simulink model "sim_localization_old"  (R2025b)
settings: Solver=ode4  StartTime=0.0  StopTime=10.0  RelTol=1e-3
values from neighbouring files (symbols this model uses):
  D = diag([0.001, 0.001, 0.0175/6, 0.0175/6, 0.0175/6, 0.0175/6*T_s, 0.0175/6*T_s].^2)    [EX_opt_1.m]    (also in init_localization.m; init_localization_template.m; script_init_localization.m)
  d = 0.165    [EX_opt_1.m]    (also in id_LEO.m; init_localization.m; init_localization_template.m; script_init_localization.m)
  d_actual = 0.164    [EX_opt_1.m]    (also in data_for_identification.mat = 0.165; init_localization.m; init_localization_template.m; script_init_localization.m)
  P_INIT_EKF = diag([0.001, 0.001, 0.0175/6, 0.0175/6, 0.0175/6, 0.0175/6*T_s, 0.0175/6*T_s].^2)    [EX_opt_1.m]    (also in init_localization.m; init_localization_template.m; script_init_localization.m)
  PHI_INIT = [0;0]    [EX_opt_1.m]    (also in data_for_identification.mat = [0 0]; id_LEO.m; init_localization.m; init_localization_template.m)
  Q_INIT = q(:,1)    [EX_opt_1.m]    (also in data_for_identification.mat = [0 0 0.463647609001]; id_LEO.m; init_localization.m = [0;0;0]; script_init_localization.m)
  r = 0.03    [EX_opt_1.m]    (also in id_LEO.m; init_localization.m; init_localization_template.m; script_init_localization.m)
  R_2 = diag([ENCODER_QUANTIZATION/6, ENCODER_QUANTIZATION/6].^2)    [EX_opt_1.m]    (also in init_localization.m = diag([ENCODER_QUANRIZATION/6,ENCODER_QUANRIZATION/6].^2); init_localization_template.m = diag([ENCODER_QUANRIZATION/6,ENCODER_QUANRIZATION/6].^2); script_init_localization.m = diag([ENCODER_QUANRIZATION/6,ENCODER_QUANRIZATION/6].^2))
  R_4 = diag([noise_std, noise_std, ENCODER_QUANTIZATION/6, ENCODER_QUANTIZATION/6].^2)    [EX_opt_1.m]    (also in init_localization.m = diag(([0.001, 0.001, ENCODER_QUANRIZATION/6,ENCODER_QUANRIZA; init_localization_template.m = diag(([0.001, 0.001, ENCODER_QUANRIZATION/6,ENCODER_QUANRIZA; script_init_localization.m = diag(([0.001, 0.001, ENCODER_QUANRIZATION/6,ENCODER_QUANRIZA)
  r_actual = 0.031    [EX_opt_1.m]    (also in data_for_identification.mat = 0.03; init_localization.m; init_localization_template.m; script_init_localization.m)
  T_s = 0.04    [EX_opt_1.m]    (also in EX_opt_2.m = Ts_values(i); data_for_identification.mat; id_LEO.m; id_template.m)
  Z_INIT_EKF = [Q_INIT_LOC; 0; 0; 0; 0]    [EX_opt_1.m]    (also in init_localization.m = [0;0;0])
settings Model: Creator=llp  LastModifiedBy=llp

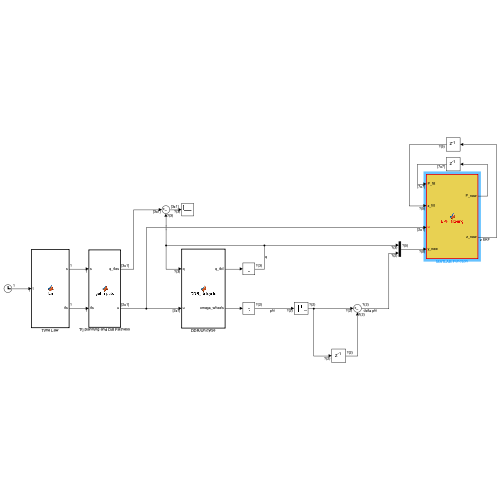
[thumbnail: Simulink's stored preview of the top-level diagram]
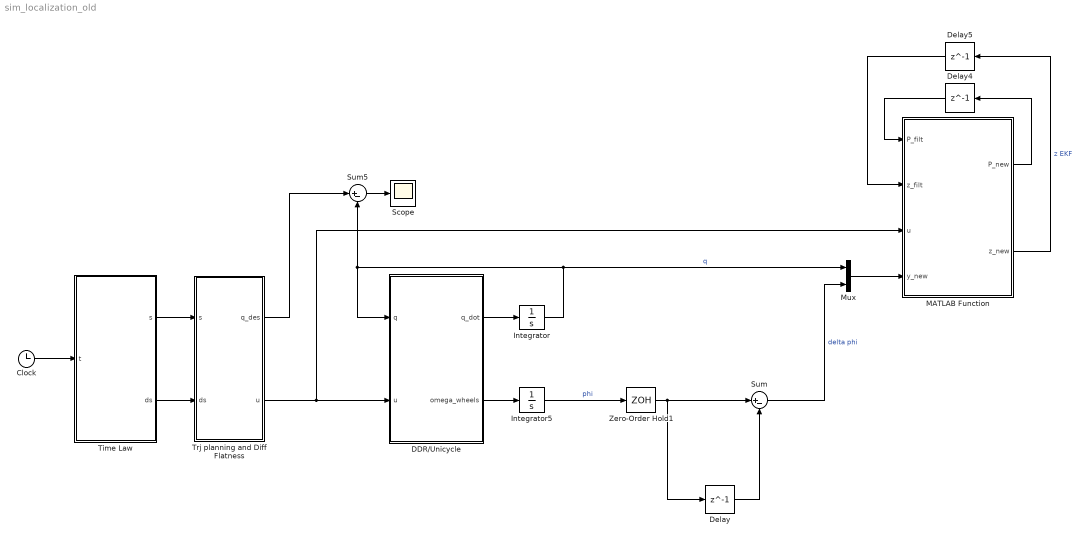
== system sim_localization_old ==
  Clock : Clock
  DDR/Unicycle : MATLAB Function  TreatAsAtomicUnit=on
  Delay : Delay  DelayLength=1  InitialCondition=[0;0]  SampleTime=T_s
  Delay4 : Delay  DelayLength=1  InitialCondition=P_INIT_EKF  SampleTime=T_s
  Delay5 : Delay  DelayLength=1  InitialCondition=Z_INIT_EKF  SampleTime=T_s
  Integrator : Integrator  InitialCondition=Q_INIT
  Integrator5 : Integrator  InitialCondition=PHI_INIT
  MATLAB Function : MATLAB Function  TreatAsAtomicUnit=on
  Mux : Mux  Inputs=2
  Scope : Scope
  Sum : Sum  Inputs=|+-
  Sum5 : Sum  Inputs=|+-
  Time Law : MATLAB Function  TreatAsAtomicUnit=on
  Trj planning and Diff Flatness : MATLAB Function  TreatAsAtomicUnit=on
  Zero-Order Hold1 : ZeroOrderHold  SampleTime=T_s
  wires:
  Integrator5/1 -> Zero-Order Hold1/1  "phi"
  Delay4/1 -> MATLAB Function/1(P_filt)
  Mux/1 -> MATLAB Function/4(y_new)
  Time Law/1(s) -> Trj planning and Diff Flatness/1(s)
  DDR/Unicycle/1(q_dot) -> Integrator/1
  Delay5/1 -> MATLAB Function/2(z_filt)
  Sum/1 -> Mux/2  "delta phi"
  Delay/1 -> Sum/2
  Sum5/1 -> Scope/1
  Integrator/1 -> Mux/1, Sum5/2, DDR/Unicycle/1(q)  "q"
  Time Law/2(ds) -> Trj planning and Diff Flatness/2(ds)
  MATLAB Function/2(z_new) -> Delay5/1  "z EKF"
  Zero-Order Hold1/1 -> Sum/1, Delay/1
  Trj planning and Diff Flatness/1(q_des) -> Sum5/1
  DDR/Unicycle/2(omega_wheels) -> Integrator5/1
  Trj planning and Diff Flatness/2(u) -> MATLAB Function/3(u), DDR/Unicycle/2(u)
  MATLAB Function/1(P_new) -> Delay4/1
  Clock/1 -> Time Law/1(t)

== matlab function sim_localization_old/Time Law ==
  data: t input; s output; ds output
function [s, ds] = fcn(t)

Ta = 0.5;
Tc = 9;

T1 = Ta;
T2 = Ta + Tc;
T3 = 2*Ta + Tc;

vc = 1/(Ta+Tc);
acc = vc/Ta;


% velocità
if t < T1
    s = 0.5*acc*t^2;
    ds = acc*t;

elseif t < T2
    s = 0.5*acc*Ta^2 + vc*(t - Ta);
    ds = vc;

elseif t < T3
    s = 0.5*acc*Ta^2 + vc*Tc + vc*(t - Ta - Tc)- 0.5*acc*(t - Ta - Tc)^2;
    ds = vc - acc*(t - Ta - Tc);

else
    s = 1;
    ds = 0;
end

== matlab function sim_localization_old/DDR//Unicycle ==
  data: q input; u input; q_dot output; omega_wheels output; d_actual parameter; r_actual parameter
function [q_dot, omega_wheels] = DDR_Unicycle(q, u, d_actual, r_actual)

theta = q(3);

v = u(1);
omega = u(2);

% ----- Cinematica unicycle -----
x_dot = v * cos(theta);
y_dot = v * sin(theta);
theta_dot = omega;

q_dot = [x_dot; y_dot; theta_dot];

% ----- Velocità ruote -----
d = d_actual;
r = r_actual;

omega_R = (v + (d/2)*omega) / r;
omega_L = (v - (d/2)*omega) / r;

omega_wheels = [omega_R; omega_L];

end

== matlab function sim_localization_old/Trj planning and Diff Flatness ==
  data: q_des output; s input; u output; ds input
function [q_des, u] = get_inputs(s, ds)

R = 0.4;
omega = 2*pi;

% ----- Traiettoria -----
x = R*sin(2*omega*s);
y = R*sin(omega*s);

% ----- Derivate rispetto a s -----
dx_s  = 2*R*omega*cos(2*omega*s);
dy_s  = R*omega*cos(omega*s);

ddx_s = -4*R*omega^2*sin(2*omega*s);
ddy_s = -R*omega^2*sin(omega*s);

% ----- Time law -----
s_dot  = ds;
s_ddot = 0;   % approx (fase a velocità costante)

% ----- Chain rule -----
dx = dx_s * s_dot;
dy = dy_s * s_dot;

ddx = ddx_s * s_dot^2 + dx_s * s_ddot;
ddy = ddy_s * s_dot^2 + dy_s * s_ddot;

% ----- Flatness -----
v = sqrt(dx^2 + dy^2);

den = dx^2 + dy^2 + 1e-6;  % evita problemi numerici
omega_u = (dx*ddy - dy*ddx) / den;

theta = atan2(dy, dx);

% ----- Output -----
q_des = [x; y; theta];
u     = [v; omega_u];

end

== matlab function sim_localization_old/MATLAB Function ==
  data: P_filt input; P_new output; z_filt input; z_new output; u input; y_new input; D parameter; R_2 parameter; R_4 parameter; T_s parameter; r parameter; d parameter
function [P_new, z_new] = EKF_filtering(P_filt, z_filt, u, y_new, D, R_2, R_4, T_s, r, d)

% ===== init output =====
z_new = zeros(3,1);
P_new = zeros(3,3);

% ===== stato =====
theta = z_filt(3);
v = u(1);
omega = u(2);

% ===== PREDICTION =====
z_pred = z_filt + T_s * [
    v*cos(theta);
    v*sin(theta);
    omega
];

% Jacobiana F
F_k = [ ...
    1, 0, -T_s*v*sin(theta);
    0, 1,  T_s*v*cos(theta);
    0, 0,  1
];

P_pred = F_k * P_filt * F_k' + D;

% ===== MEASUREMENT =====
% esempio: misura diretta stato
H_k = eye(3);

y_pred = z_pred;

e = y_new - y_pred;

R = blkdiag(R_2, R_4);

% ===== UPDATE =====
K = P_pred * H_k' / (H_k * P_pred * H_k' + R);

z_new = z_pred + K * e;

P_new = P_pred - K * H_k * P_pred;

end
